simulink model "DTU_Topology_Rural"  (R2023b)
settings: Solver=ode4  StartTime=0.0  StopTime=stoptime  FixedStep=Ts  RelTol=1e-3
PreLoadFcn:
  | Ts=1e-4;load('RuralCase_11052022_12052022_Data_with_ParThreads_Final.mat');run('line_parameters.m');run('Grid_Parameters_3ph.m');
PostLoadFcn:
  | Ts=1e-4;load('RuralCase_11052022_12052022_Data_with_ParThreads_Final.mat');run('line_parameters.m');run('Grid_Parameters_3ph.m');
InitFcn:
  | Ts=1e-4;load('RuralCase_11052022_12052022_Data_with_ParThreads_Final.mat');run('line_parameters.m');run('Grid_Parameters_3ph.m');
StartFcn:
  | Ts=1e-4;load('RuralCase_11052022_12052022_Data_with_ParThreads_Final.mat');run('line_parameters.m');run('Grid_Parameters_3ph.m');
values from neighbouring files (symbols this model uses):
  datastart = 1    [Grid_Parameters_3ph.m]
  datastop = 21556    [Grid_Parameters_3ph.m]
  DTUsignconv = -1000    [Grid_Parameters_3ph.m]
  fnom = 50    [Grid_Parameters_3ph.m]    (also in line_parameters.m)
  line_param = struct()    [line_parameters.m]
  Time = cumsum([0;ones(stoptime,1)])    [Grid_Parameters_3ph.m]
  timestep_meas_data = 1    [Grid_Parameters_3ph.m]
  Vnom = 400    [Grid_Parameters_3ph.m]
undefined symbols (not defined in the file or in its folder): another_event_name, data, j, my_event_name, Newton, Raphson, t_factor
libraries: spsSeriesRLCBranchLib x126, spsGroundLib x71, spsThreePhaseSineGeneratorLib x42, spsControlledCurrentSourceLib x39, spsThreePhaseVIMeasurementLib x26, spsMeanLib x24, spsPowerLib x14, spsMutualInductanceLib x7, rtlab x3, powerlib_meascontrol x3, spsControlledVoltageSourceLib x3, spsThreePhaseSourceLib x1
(part 2 of 5)

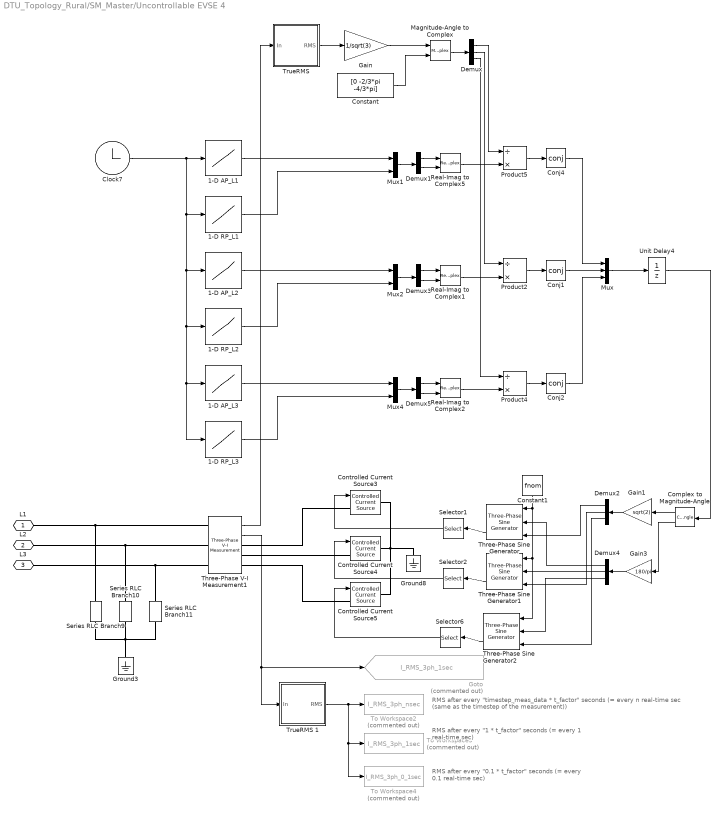
== system DTU_Topology_Rural/SM_Master/Uncontrollable EVSE 4 ==
  note: RMS after every "1 * t_factor" seconds
      | (= every 1 real-time sec)
  note: RMS after every "0.1 * t_factor" seconds
      | (= every 0.1 real-time sec)
  note: RMS after every "timestep_meas_data * t_factor" seconds
      | (= every n real-time sec (same as the timestep of the measurement))
  1-D AP_L1 : Lookup_n-D  NumberOfTableDimensions=1  BreakpointsForDimension1=Time  Table="data.(\"117-6_NEVIC4_phaseA_ActivePower\")(datastart:datastop) * DTUsignconv"  InterpMethod=Flat  InternalRulePriority=Speed  RndMeth=Simplest
  1-D AP_L2 : Lookup_n-D  NumberOfTableDimensions=1  BreakpointsForDimension1=Time  Table="data.(\"117-6_NEVIC4_phaseB_ActivePower\")(datastart:datastop) * DTUsignconv"  InterpMethod=Flat  InternalRulePriority=Speed  RndMeth=Simplest
  1-D AP_L3 : Lookup_n-D  NumberOfTableDimensions=1  BreakpointsForDimension1=Time  Table="data.(\"117-6_NEVIC4_phaseC_ActivePower\")(datastart:datastop) * DTUsignconv"  InterpMethod=Flat  InternalRulePriority=Speed  RndMeth=Simplest
  1-D RP_L1 : Lookup_n-D  NumberOfTableDimensions=1  BreakpointsForDimension1=Time  Table="data.(\"117-6_NEVIC4_phaseA_ReactivePower\")(datastart:datastop) * DTUsignconv"  InterpMethod=Flat  InternalRulePriority=Speed  RndMeth=Simplest
  1-D RP_L2 : Lookup_n-D  NumberOfTableDimensions=1  BreakpointsForDimension1=Time  Table="data.(\"117-6_NEVIC4_phaseB_ReactivePower\")(datastart:datastop) * DTUsignconv"  InterpMethod=Flat  InternalRulePriority=Speed  RndMeth=Simplest
  1-D RP_L3 : Lookup_n-D  NumberOfTableDimensions=1  BreakpointsForDimension1=Time  Table="data.(\"117-6_NEVIC4_phaseC_ReactivePower\")(datastart:datastop) * DTUsignconv"  InterpMethod=Flat  InternalRulePriority=Speed  RndMeth=Simplest
  Clock7 : Clock
  Complex to Magnitude-Angle : ComplexToMagnitudeAngle
  Conj1 : Math  Operator=conj  SignedPower=on
  Conj2 : Math  Operator=conj  SignedPower=on
  Conj4 : Math  Operator=conj  SignedPower=on
  Constant : Constant  Value=[0 -2/3*pi -4/3*pi]
  Constant1 : Constant  Value=fnom
  Controlled Current Source3 : spsControlledCurrentSourceLib/Controlled Current Source  Initialize=on  Source_Type=AC  Amplitude=0  Phase=0  Frequency=50  Measurements=Current
  Controlled Current Source4 : spsControlledCurrentSourceLib/Controlled Current Source  Initialize=on  Source_Type=AC  Amplitude=0  Phase=0  Frequency=50  Measurements=Current
  Controlled Current Source5 : spsControlledCurrentSourceLib/Controlled Current Source  Initialize=on  Source_Type=AC  Amplitude=0  Phase=0  Frequency=50  Measurements=Current
  Demux : Demux  Outputs=3
  Demux1 : Demux  Outputs=2
      settings: DisplayOption=none
  Demux2 : Demux  Outputs=3
  Demux3 : Demux  Outputs=2
      settings: DisplayOption=none
  Demux4 : Demux  Outputs=3
  Demux5 : Demux  Outputs=2
      settings: DisplayOption=none
  Gain : Gain  Gain=1/sqrt(3)
  Gain1 : Gain  Gain=sqrt(2)
  Gain3 : Gain  Gain=180/pi
  Goto : Goto  Commented=on  GotoTag=I_RMS_3ph_1sec  TagVisibility=global
  Ground3 : spsGroundLib/Ground  LConnTagsString=a
  Ground8 : spsGroundLib/Ground  LConnTagsString=a
  Magnitude-Angle to Complex : MagnitudeAngleToComplex
  Mux : Mux  Inputs=3
  Mux1 : Mux  Inputs=2
  Mux2 : Mux  Inputs=2
  Mux4 : Mux  Inputs=2
  Product2 : Product  Inputs=/*  InputSameDT=on  SaturateOnIntegerOverflow=on  OutDataTypeStr=Inherit: Same as first input
  Product4 : Product  Inputs=/*  InputSameDT=on  SaturateOnIntegerOverflow=on  OutDataTypeStr=Inherit: Same as first input
  Product5 : Product  Inputs=/*  InputSameDT=on  SaturateOnIntegerOverflow=on  OutDataTypeStr=Inherit: Same as first input
  Real-Imag to Complex1 : RealImagToComplex
  Real-Imag to Complex2 : RealImagToComplex
  Real-Imag to Complex5 : RealImagToComplex
  Selector1 : Selector  InputPortWidth=3  IndexOptions=Index vector (dialog)  Indices=1  OutputSizes=1
  Selector2 : Selector  InputPortWidth=3  IndexOptions=Index vector (dialog)  Indices=1  OutputSizes=1
  Selector6 : Selector  InputPortWidth=3  IndexOptions=Index vector (dialog)  Indices=1  OutputSizes=1
  Series RLC Branch10 : spsSeriesRLCBranchLib/Series RLC Branch  LConnTagsString=__new0  RConnTagsString=__new0  BranchType=R  Resistance=1e12  Inductance=1e-3  SetiL0=off  InitialCurrent=0  Capacitance=1e-6  Setx0=off  InitialVoltage=0  Measurements=None
  Series RLC Branch11 : spsSeriesRLCBranchLib/Series RLC Branch  LConnTagsString=__new0  RConnTagsString=__new0  BranchType=R  Resistance=1e12  Inductance=1e-3  SetiL0=off  InitialCurrent=0  Capacitance=1e-6  Setx0=off  InitialVoltage=0  Measurements=None
  Series RLC Branch9 : spsSeriesRLCBranchLib/Series RLC Branch  LConnTagsString=__new0  RConnTagsString=__new0  BranchType=R  Resistance=1e12  Inductance=1e-3  SetiL0=off  InitialCurrent=0  Capacitance=1e-6  Setx0=off  InitialVoltage=0  Measurements=None
  Three-Phase Sine Generator : spsThreePhaseSineGeneratorLib/Three-Phase Sine Generator  Ts=0
      settings: LibrarySourceBlock=|
      | sps_lib/Sources/Signal Generator Sources/Three-Phase
      | Sine Generator
  Three-Phase Sine Generator1 : spsThreePhaseSineGeneratorLib/Three-Phase Sine Generator  Ts=0
      settings: LibrarySourceBlock=|
      | sps_lib/Sources/Signal Generator Sources/Three-Phase
      | Sine Generator
  Three-Phase Sine Generator2 : spsThreePhaseSineGeneratorLib/Three-Phase Sine Generator  Ts=0
      settings: LibrarySourceBlock=|
      | sps_lib/Sources/Signal Generator Sources/Three-Phase
      | Sine Generator
  Three-Phase V-I Measurement1 : spsThreePhaseVIMeasurementLib/Three-Phase V-I Measurement  VoltageMeasurement=phase-to-phase  SetLabelV=off  LabelV=Vabc  Vpu=off  VpuLL=off  CurrentMeasurement=yes  SetLabelI=off  LabelI=Iabc  Ipu=off  Pbase=100e6  Vbase=Vnom*sqrt(3)  OutputType=Complex  PhasorSimulation=off  PSBequivalent=0
  To Workspace2 : ToWorkspace  Commented=on  VariableName=I_RMS_3ph_nsec  SampleTime=timestep_meas_data * t_factor
  To Workspace4 : ToWorkspace  Commented=on  VariableName=I_RMS_3ph_0_1sec  SampleTime=0.1 * t_factor
  To Workspace5 : ToWorkspace  Commented=on  VariableName=I_RMS_3ph_1sec  SampleTime=1 * t_factor
  "TrueRMS " : Subsystem  AncestorBlock=powerlib_meascontrol/Measurements/RMS/TrueRMS
  TrueRMS 1 : Subsystem  AncestorBlock=powerlib_meascontrol/Measurements/RMS/TrueRMS
  Unit Delay4 : UnitDelay  InitialCondition=0*exp(-j*0*pi/180)  SampleTime=Ts  HasFrameUpgradeWarning=on
  L1 : PMIOPort  Side=Right
  L2 : PMIOPort  Port=2  Side=Right
  L3 : PMIOPort  Port=3  Side=Right
  wires:
  1-D AP_L1/1 -> Mux1/1
  Product5/1 -> Conj4/1
  Three-Phase V-I Measurement1/2 -> Goto/1, TrueRMS 1/1(In)
  Mux1/1 -> Demux1/1
  Real-Imag to Complex5/1 -> Product5/2
  Clock7/1 -> 1-D RP_L1/1, 1-D RP_L2/1, 1-D AP_L3/1, 1-D RP_L3/1, 1-D AP_L2/1, 1-D AP_L1/1
  TrueRMS 1/1(RMS) -> To Workspace2/1, To Workspace5/1, To Workspace4/1
  Constant/1 -> Magnitude-Angle to Complex/2
  Demux/1 -> Product5/1
  Demux/2 -> Product2/1
  Demux/3 -> Product4/1
  Magnitude-Angle to Complex/1 -> Demux/1
  Gain/1 -> Magnitude-Angle to Complex/1
  Mux/1 -> Unit Delay4/1
  Complex to Magnitude-Angle/1 -> Gain1/1
  Three-Phase Sine Generator/1 -> Selector1/1
  Three-Phase Sine Generator1/1 -> Selector2/1
  Three-Phase Sine Generator2/1 -> Selector6/1
  Selector2/1 -> Controlled Current Source4/1
  Selector6/1 -> Controlled Current Source5/1
  Demux2/1 -> Three-Phase Sine Generator/1
  Demux2/2 -> Three-Phase Sine Generator1/1
  Demux2/3 -> Three-Phase Sine Generator2/1
  Conj4/1 -> Mux/1
  Conj1/1 -> Mux/2
  Conj2/1 -> Mux/3
  Constant1/1 -> Three-Phase Sine Generator/3, Three-Phase Sine Generator2/3, Three-Phase Sine Generator1/3
  Complex to Magnitude-Angle/2 -> Gain3/1
  Gain3/1 -> Demux4/1
  Selector1/1 -> Controlled Current Source3/1
  Demux4/1 -> Three-Phase Sine Generator/2
  Demux4/2 -> Three-Phase Sine Generator1/2
  Demux4/3 -> Three-Phase Sine Generator2/2
  Gain1/1 -> Demux2/1
  Demux1/1 -> Real-Imag to Complex5/1
  Demux1/2 -> Real-Imag to Complex5/2
  "TrueRMS "/1(RMS) -> Gain/1
  Three-Phase V-I Measurement1/1 -> "TrueRMS "/1(In)
  Unit Delay4/1 -> Complex to Magnitude-Angle/1
  Mux2/1 -> Demux3/1
  Demux3/2 -> Real-Imag to Complex1/2
  Real-Imag to Complex1/1 -> Product2/2
  Demux3/1 -> Real-Imag to Complex1/1
  1-D AP_L2/1 -> Mux2/1
  Product2/1 -> Conj1/1
  Mux4/1 -> Demux5/1
  Demux5/2 -> Real-Imag to Complex2/2
  Real-Imag to Complex2/1 -> Product4/2
  Demux5/1 -> Real-Imag to Complex2/1
  1-D AP_L3/1 -> Mux4/1
  Product4/1 -> Conj2/1
  1-D RP_L1/1 -> Mux1/2
  1-D RP_L2/1 -> Mux2/2
  1-D RP_L3/1 -> Mux4/2
  connections:
  Three-Phase V-I Measurement1/RConn2 -- Controlled Current Source4/LConn1
  Three-Phase V-I Measurement1/RConn1 -- Controlled Current Source3/LConn1
  Three-Phase V-I Measurement1/RConn3 -- Controlled Current Source5/LConn1
  Controlled Current Source3/RConn1 -- Controlled Current Source4/RConn1 -- Ground8/LConn1 -- Controlled Current Source5/RConn1
  L1/RConn1 -- Three-Phase V-I Measurement1/LConn1 -- Series RLC Branch9/LConn1
  Series RLC Branch10/LConn1 -- Three-Phase V-I Measurement1/LConn2 -- L2/RConn1
  Series RLC Branch11/LConn1 -- Three-Phase V-I Measurement1/LConn3 -- L3/RConn1
  Series RLC Branch9/RConn1 -- Series RLC Branch10/RConn1 -- Ground3/LConn1 -- Series RLC Branch11/RConn1

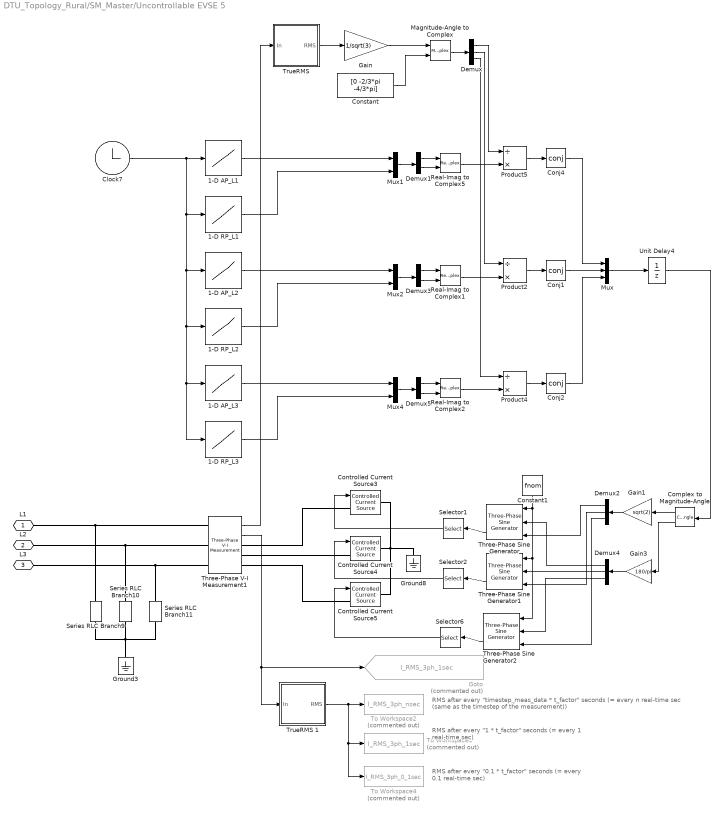
== system DTU_Topology_Rural/SM_Master/Uncontrollable EVSE 5 ==
  note: RMS after every "1 * t_factor" seconds
      | (= every 1 real-time sec)
  note: RMS after every "0.1 * t_factor" seconds
      | (= every 0.1 real-time sec)
  note: RMS after every "timestep_meas_data * t_factor" seconds
      | (= every n real-time sec (same as the timestep of the measurement))
  1-D AP_L1 : Lookup_n-D  NumberOfTableDimensions=1  BreakpointsForDimension1=Time  Table="data.(\"117-6_NEVIC5_phaseA_ActivePower\")(datastart:datastop) * DTUsignconv"  InterpMethod=Flat  InternalRulePriority=Speed  RndMeth=Simplest
  1-D AP_L2 : Lookup_n-D  NumberOfTableDimensions=1  BreakpointsForDimension1=Time  Table="data.(\"117-6_NEVIC5_phaseB_ActivePower\")(datastart:datastop) * DTUsignconv"  InterpMethod=Flat  InternalRulePriority=Speed  RndMeth=Simplest
  1-D AP_L3 : Lookup_n-D  NumberOfTableDimensions=1  BreakpointsForDimension1=Time  Table="data.(\"117-6_NEVIC5_phaseC_ActivePower\")(datastart:datastop) * DTUsignconv"  InterpMethod=Flat  InternalRulePriority=Speed  RndMeth=Simplest
  1-D RP_L1 : Lookup_n-D  NumberOfTableDimensions=1  BreakpointsForDimension1=Time  Table="data.(\"117-6_NEVIC5_phaseA_ReactivePower\")(datastart:datastop) * DTUsignconv"  InterpMethod=Flat  InternalRulePriority=Speed  RndMeth=Simplest
  1-D RP_L2 : Lookup_n-D  NumberOfTableDimensions=1  BreakpointsForDimension1=Time  Table="data.(\"117-6_NEVIC5_phaseB_ReactivePower\")(datastart:datastop) * DTUsignconv"  InterpMethod=Flat  InternalRulePriority=Speed  RndMeth=Simplest
  1-D RP_L3 : Lookup_n-D  NumberOfTableDimensions=1  BreakpointsForDimension1=Time  Table="data.(\"117-6_NEVIC5_phaseC_ReactivePower\")(datastart:datastop) * DTUsignconv"  InterpMethod=Flat  InternalRulePriority=Speed  RndMeth=Simplest
  Clock7 : Clock
  Complex to Magnitude-Angle : ComplexToMagnitudeAngle
  Conj1 : Math  Operator=conj  SignedPower=on
  Conj2 : Math  Operator=conj  SignedPower=on
  Conj4 : Math  Operator=conj  SignedPower=on
  Constant : Constant  Value=[0 -2/3*pi -4/3*pi]
  Constant1 : Constant  Value=fnom
  Controlled Current Source3 : spsControlledCurrentSourceLib/Controlled Current Source  Initialize=on  Source_Type=AC  Amplitude=0  Phase=0  Frequency=50  Measurements=Current
  Controlled Current Source4 : spsControlledCurrentSourceLib/Controlled Current Source  Initialize=on  Source_Type=AC  Amplitude=0  Phase=0  Frequency=50  Measurements=Current
  Controlled Current Source5 : spsControlledCurrentSourceLib/Controlled Current Source  Initialize=on  Source_Type=AC  Amplitude=0  Phase=0  Frequency=50  Measurements=Current
  Demux : Demux  Outputs=3
  Demux1 : Demux  Outputs=2
      settings: DisplayOption=none
  Demux2 : Demux  Outputs=3
  Demux3 : Demux  Outputs=2
      settings: DisplayOption=none
  Demux4 : Demux  Outputs=3
  Demux5 : Demux  Outputs=2
      settings: DisplayOption=none
  Gain : Gain  Gain=1/sqrt(3)
  Gain1 : Gain  Gain=sqrt(2)
  Gain3 : Gain  Gain=180/pi
  Goto : Goto  Commented=on  GotoTag=I_RMS_3ph_1sec  TagVisibility=global
  Ground3 : spsGroundLib/Ground  LConnTagsString=a
  Ground8 : spsGroundLib/Ground  LConnTagsString=a
  Magnitude-Angle to Complex : MagnitudeAngleToComplex
  Mux : Mux  Inputs=3
  Mux1 : Mux  Inputs=2
  Mux2 : Mux  Inputs=2
  Mux4 : Mux  Inputs=2
  Product2 : Product  Inputs=/*  InputSameDT=on  SaturateOnIntegerOverflow=on  OutDataTypeStr=Inherit: Same as first input
  Product4 : Product  Inputs=/*  InputSameDT=on  SaturateOnIntegerOverflow=on  OutDataTypeStr=Inherit: Same as first input
  Product5 : Product  Inputs=/*  InputSameDT=on  SaturateOnIntegerOverflow=on  OutDataTypeStr=Inherit: Same as first input
  Real-Imag to Complex1 : RealImagToComplex
  Real-Imag to Complex2 : RealImagToComplex
  Real-Imag to Complex5 : RealImagToComplex
  Selector1 : Selector  InputPortWidth=3  IndexOptions=Index vector (dialog)  Indices=1  OutputSizes=1
  Selector2 : Selector  InputPortWidth=3  IndexOptions=Index vector (dialog)  Indices=1  OutputSizes=1
  Selector6 : Selector  InputPortWidth=3  IndexOptions=Index vector (dialog)  Indices=1  OutputSizes=1
  Series RLC Branch10 : spsSeriesRLCBranchLib/Series RLC Branch  LConnTagsString=__new0  RConnTagsString=__new0  BranchType=R  Resistance=1e12  Inductance=1e-3  SetiL0=off  InitialCurrent=0  Capacitance=1e-6  Setx0=off  InitialVoltage=0  Measurements=None
  Series RLC Branch11 : spsSeriesRLCBranchLib/Series RLC Branch  LConnTagsString=__new0  RConnTagsString=__new0  BranchType=R  Resistance=1e12  Inductance=1e-3  SetiL0=off  InitialCurrent=0  Capacitance=1e-6  Setx0=off  InitialVoltage=0  Measurements=None
  Series RLC Branch9 : spsSeriesRLCBranchLib/Series RLC Branch  LConnTagsString=__new0  RConnTagsString=__new0  BranchType=R  Resistance=1e12  Inductance=1e-3  SetiL0=off  InitialCurrent=0  Capacitance=1e-6  Setx0=off  InitialVoltage=0  Measurements=None
  Three-Phase Sine Generator : spsThreePhaseSineGeneratorLib/Three-Phase Sine Generator  Ts=0
      settings: LibrarySourceBlock=|
      | sps_lib/Sources/Signal Generator Sources/Three-Phase
      | Sine Generator
  Three-Phase Sine Generator1 : spsThreePhaseSineGeneratorLib/Three-Phase Sine Generator  Ts=0
      settings: LibrarySourceBlock=|
      | sps_lib/Sources/Signal Generator Sources/Three-Phase
      | Sine Generator
  Three-Phase Sine Generator2 : spsThreePhaseSineGeneratorLib/Three-Phase Sine Generator  Ts=0
      settings: LibrarySourceBlock=|
      | sps_lib/Sources/Signal Generator Sources/Three-Phase
      | Sine Generator
  Three-Phase V-I Measurement1 : spsThreePhaseVIMeasurementLib/Three-Phase V-I Measurement  VoltageMeasurement=phase-to-phase  SetLabelV=off  LabelV=Vabc  Vpu=off  VpuLL=off  CurrentMeasurement=yes  SetLabelI=off  LabelI=Iabc  Ipu=off  Pbase=100e6  Vbase=Vnom*sqrt(3)  OutputType=Complex  PhasorSimulation=off  PSBequivalent=0
  To Workspace2 : ToWorkspace  Commented=on  VariableName=I_RMS_3ph_nsec  SampleTime=timestep_meas_data * t_factor
  To Workspace4 : ToWorkspace  Commented=on  VariableName=I_RMS_3ph_0_1sec  SampleTime=0.1 * t_factor
  To Workspace5 : ToWorkspace  Commented=on  VariableName=I_RMS_3ph_1sec  SampleTime=1 * t_factor
  "TrueRMS " : Subsystem  AncestorBlock=powerlib_meascontrol/Measurements/RMS/TrueRMS
  TrueRMS 1 : Subsystem  AncestorBlock=powerlib_meascontrol/Measurements/RMS/TrueRMS
  Unit Delay4 : UnitDelay  InitialCondition=0*exp(-j*0*pi/180)  SampleTime=Ts  HasFrameUpgradeWarning=on
  L1 : PMIOPort  Side=Right
  L2 : PMIOPort  Port=2  Side=Right
  L3 : PMIOPort  Port=3  Side=Right
  wires:
  1-D AP_L1/1 -> Mux1/1
  Product5/1 -> Conj4/1
  Three-Phase V-I Measurement1/2 -> Goto/1, TrueRMS 1/1(In)
  Mux1/1 -> Demux1/1
  Real-Imag to Complex5/1 -> Product5/2
  Clock7/1 -> 1-D RP_L1/1, 1-D RP_L2/1, 1-D AP_L3/1, 1-D RP_L3/1, 1-D AP_L2/1, 1-D AP_L1/1
  TrueRMS 1/1(RMS) -> To Workspace2/1, To Workspace5/1, To Workspace4/1
  Constant/1 -> Magnitude-Angle to Complex/2
  Demux/1 -> Product5/1
  Demux/2 -> Product2/1
  Demux/3 -> Product4/1
  Magnitude-Angle to Complex/1 -> Demux/1
  Gain/1 -> Magnitude-Angle to Complex/1
  Mux/1 -> Unit Delay4/1
  Complex to Magnitude-Angle/1 -> Gain1/1
  Three-Phase Sine Generator/1 -> Selector1/1
  Three-Phase Sine Generator1/1 -> Selector2/1
  Three-Phase Sine Generator2/1 -> Selector6/1
  Selector2/1 -> Controlled Current Source4/1
  Selector6/1 -> Controlled Current Source5/1
  Demux2/1 -> Three-Phase Sine Generator/1
  Demux2/2 -> Three-Phase Sine Generator1/1
  Demux2/3 -> Three-Phase Sine Generator2/1
  Conj4/1 -> Mux/1
  Conj1/1 -> Mux/2
  Conj2/1 -> Mux/3
  Constant1/1 -> Three-Phase Sine Generator/3, Three-Phase Sine Generator2/3, Three-Phase Sine Generator1/3
  Complex to Magnitude-Angle/2 -> Gain3/1
  Gain3/1 -> Demux4/1
  Selector1/1 -> Controlled Current Source3/1
  Demux4/1 -> Three-Phase Sine Generator/2
  Demux4/2 -> Three-Phase Sine Generator1/2
  Demux4/3 -> Three-Phase Sine Generator2/2
  Gain1/1 -> Demux2/1
  Demux1/1 -> Real-Imag to Complex5/1
  Demux1/2 -> Real-Imag to Complex5/2
  "TrueRMS "/1(RMS) -> Gain/1
  Three-Phase V-I Measurement1/1 -> "TrueRMS "/1(In)
  Unit Delay4/1 -> Complex to Magnitude-Angle/1
  Mux2/1 -> Demux3/1
  Demux3/2 -> Real-Imag to Complex1/2
  Real-Imag to Complex1/1 -> Product2/2
  Demux3/1 -> Real-Imag to Complex1/1
  1-D AP_L2/1 -> Mux2/1
  Product2/1 -> Conj1/1
  Mux4/1 -> Demux5/1
  Demux5/2 -> Real-Imag to Complex2/2
  Real-Imag to Complex2/1 -> Product4/2
  Demux5/1 -> Real-Imag to Complex2/1
  1-D AP_L3/1 -> Mux4/1
  Product4/1 -> Conj2/1
  1-D RP_L1/1 -> Mux1/2
  1-D RP_L2/1 -> Mux2/2
  1-D RP_L3/1 -> Mux4/2
  connections:
  Three-Phase V-I Measurement1/RConn2 -- Controlled Current Source4/LConn1
  Three-Phase V-I Measurement1/RConn1 -- Controlled Current Source3/LConn1
  Three-Phase V-I Measurement1/RConn3 -- Controlled Current Source5/LConn1
  Controlled Current Source3/RConn1 -- Controlled Current Source4/RConn1 -- Ground8/LConn1 -- Controlled Current Source5/RConn1
  L1/RConn1 -- Three-Phase V-I Measurement1/LConn1 -- Series RLC Branch9/LConn1
  Series RLC Branch10/LConn1 -- Three-Phase V-I Measurement1/LConn2 -- L2/RConn1
  Series RLC Branch11/LConn1 -- Three-Phase V-I Measurement1/LConn3 -- L3/RConn1
  Series RLC Branch9/RConn1 -- Series RLC Branch10/RConn1 -- Ground3/LConn1 -- Series RLC Branch11/RConn1

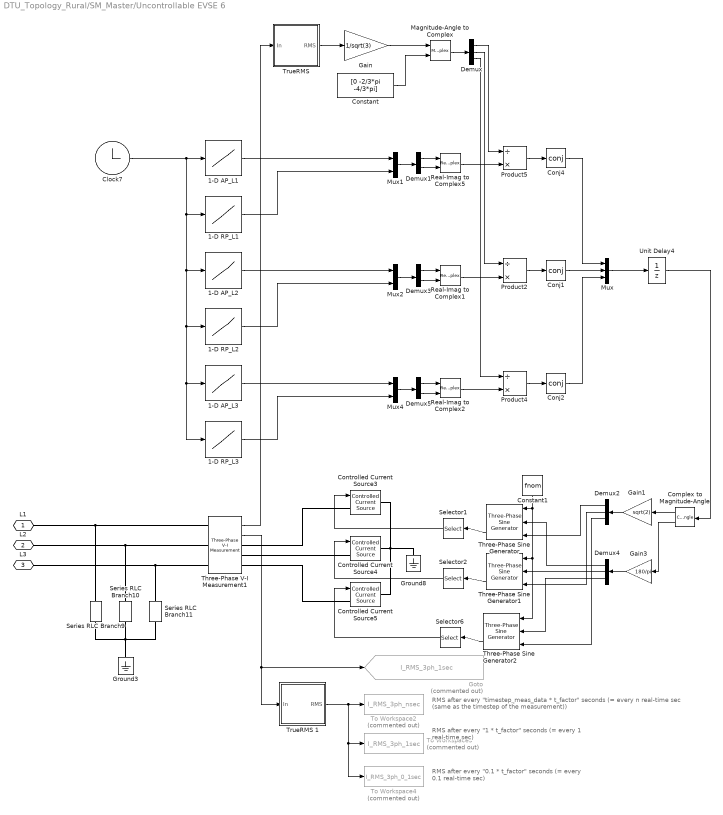
== system DTU_Topology_Rural/SM_Master/Uncontrollable EVSE 6 ==
  note: RMS after every "1 * t_factor" seconds
      | (= every 1 real-time sec)
  note: RMS after every "0.1 * t_factor" seconds
      | (= every 0.1 real-time sec)
  note: RMS after every "timestep_meas_data * t_factor" seconds
      | (= every n real-time sec (same as the timestep of the measurement))
  1-D AP_L1 : Lookup_n-D  NumberOfTableDimensions=1  BreakpointsForDimension1=Time  Table="data.(\"117-6_NEVIC6_phaseA_ActivePower\")(datastart:datastop) * DTUsignconv"  InterpMethod=Flat  InternalRulePriority=Speed  RndMeth=Simplest
  1-D AP_L2 : Lookup_n-D  NumberOfTableDimensions=1  BreakpointsForDimension1=Time  Table="data.(\"117-6_NEVIC6_phaseB_ActivePower\")(datastart:datastop) * DTUsignconv"  InterpMethod=Flat  InternalRulePriority=Speed  RndMeth=Simplest
  1-D AP_L3 : Lookup_n-D  NumberOfTableDimensions=1  BreakpointsForDimension1=Time  Table="data.(\"117-6_NEVIC6_phaseC_ActivePower\")(datastart:datastop) * DTUsignconv"  InterpMethod=Flat  InternalRulePriority=Speed  RndMeth=Simplest
  1-D RP_L1 : Lookup_n-D  NumberOfTableDimensions=1  BreakpointsForDimension1=Time  Table="data.(\"117-6_NEVIC6_phaseA_ReactivePower\")(datastart:datastop) * DTUsignconv"  InterpMethod=Flat  InternalRulePriority=Speed  RndMeth=Simplest
  1-D RP_L2 : Lookup_n-D  NumberOfTableDimensions=1  BreakpointsForDimension1=Time  Table="data.(\"117-6_NEVIC6_phaseB_ReactivePower\")(datastart:datastop) * DTUsignconv"  InterpMethod=Flat  InternalRulePriority=Speed  RndMeth=Simplest
  1-D RP_L3 : Lookup_n-D  NumberOfTableDimensions=1  BreakpointsForDimension1=Time  Table="data.(\"117-6_NEVIC6_phaseC_ReactivePower\")(datastart:datastop) * DTUsignconv"  InterpMethod=Flat  InternalRulePriority=Speed  RndMeth=Simplest
  Clock7 : Clock
  Complex to Magnitude-Angle : ComplexToMagnitudeAngle
  Conj1 : Math  Operator=conj  SignedPower=on
  Conj2 : Math  Operator=conj  SignedPower=on
  Conj4 : Math  Operator=conj  SignedPower=on
  Constant : Constant  Value=[0 -2/3*pi -4/3*pi]
  Constant1 : Constant  Value=fnom
  Controlled Current Source3 : spsControlledCurrentSourceLib/Controlled Current Source  Initialize=on  Source_Type=AC  Amplitude=0  Phase=0  Frequency=50  Measurements=Current
  Controlled Current Source4 : spsControlledCurrentSourceLib/Controlled Current Source  Initialize=on  Source_Type=AC  Amplitude=0  Phase=0  Frequency=50  Measurements=Current
  Controlled Current Source5 : spsControlledCurrentSourceLib/Controlled Current Source  Initialize=on  Source_Type=AC  Amplitude=0  Phase=0  Frequency=50  Measurements=Current
  Demux : Demux  Outputs=3
  Demux1 : Demux  Outputs=2
      settings: DisplayOption=none
  Demux2 : Demux  Outputs=3
  Demux3 : Demux  Outputs=2
      settings: DisplayOption=none
  Demux4 : Demux  Outputs=3
  Demux5 : Demux  Outputs=2
      settings: DisplayOption=none
  Gain : Gain  Gain=1/sqrt(3)
  Gain1 : Gain  Gain=sqrt(2)
  Gain3 : Gain  Gain=180/pi
  Goto : Goto  Commented=on  GotoTag=I_RMS_3ph_1sec  TagVisibility=global
  Ground3 : spsGroundLib/Ground  LConnTagsString=a
  Ground8 : spsGroundLib/Ground  LConnTagsString=a
  Magnitude-Angle to Complex : MagnitudeAngleToComplex
  Mux : Mux  Inputs=3
  Mux1 : Mux  Inputs=2
  Mux2 : Mux  Inputs=2
  Mux4 : Mux  Inputs=2
  Product2 : Product  Inputs=/*  InputSameDT=on  SaturateOnIntegerOverflow=on  OutDataTypeStr=Inherit: Same as first input
  Product4 : Product  Inputs=/*  InputSameDT=on  SaturateOnIntegerOverflow=on  OutDataTypeStr=Inherit: Same as first input
  Product5 : Product  Inputs=/*  InputSameDT=on  SaturateOnIntegerOverflow=on  OutDataTypeStr=Inherit: Same as first input
  Real-Imag to Complex1 : RealImagToComplex
  Real-Imag to Complex2 : RealImagToComplex
  Real-Imag to Complex5 : RealImagToComplex
  Selector1 : Selector  InputPortWidth=3  IndexOptions=Index vector (dialog)  Indices=1  OutputSizes=1
  Selector2 : Selector  InputPortWidth=3  IndexOptions=Index vector (dialog)  Indices=1  OutputSizes=1
  Selector6 : Selector  InputPortWidth=3  IndexOptions=Index vector (dialog)  Indices=1  OutputSizes=1
  Series RLC Branch10 : spsSeriesRLCBranchLib/Series RLC Branch  LConnTagsString=__new0  RConnTagsString=__new0  BranchType=R  Resistance=1e12  Inductance=1e-3  SetiL0=off  InitialCurrent=0  Capacitance=1e-6  Setx0=off  InitialVoltage=0  Measurements=None
  Series RLC Branch11 : spsSeriesRLCBranchLib/Series RLC Branch  LConnTagsString=__new0  RConnTagsString=__new0  BranchType=R  Resistance=1e12  Inductance=1e-3  SetiL0=off  InitialCurrent=0  Capacitance=1e-6  Setx0=off  InitialVoltage=0  Measurements=None
  Series RLC Branch9 : spsSeriesRLCBranchLib/Series RLC Branch  LConnTagsString=__new0  RConnTagsString=__new0  BranchType=R  Resistance=1e12  Inductance=1e-3  SetiL0=off  InitialCurrent=0  Capacitance=1e-6  Setx0=off  InitialVoltage=0  Measurements=None
  Three-Phase Sine Generator : spsThreePhaseSineGeneratorLib/Three-Phase Sine Generator  Ts=0
      settings: LibrarySourceBlock=|
      | sps_lib/Sources/Signal Generator Sources/Three-Phase
      | Sine Generator
  Three-Phase Sine Generator1 : spsThreePhaseSineGeneratorLib/Three-Phase Sine Generator  Ts=0
      settings: LibrarySourceBlock=|
      | sps_lib/Sources/Signal Generator Sources/Three-Phase
      | Sine Generator
  Three-Phase Sine Generator2 : spsThreePhaseSineGeneratorLib/Three-Phase Sine Generator  Ts=0
      settings: LibrarySourceBlock=|
      | sps_lib/Sources/Signal Generator Sources/Three-Phase
      | Sine Generator
  Three-Phase V-I Measurement1 : spsThreePhaseVIMeasurementLib/Three-Phase V-I Measurement  VoltageMeasurement=phase-to-phase  SetLabelV=off  LabelV=Vabc  Vpu=off  VpuLL=off  CurrentMeasurement=yes  SetLabelI=off  LabelI=Iabc  Ipu=off  Pbase=100e6  Vbase=Vnom*sqrt(3)  OutputType=Complex  PhasorSimulation=off  PSBequivalent=0
  To Workspace2 : ToWorkspace  Commented=on  VariableName=I_RMS_3ph_nsec  SampleTime=timestep_meas_data * t_factor
  To Workspace4 : ToWorkspace  Commented=on  VariableName=I_RMS_3ph_0_1sec  SampleTime=0.1 * t_factor
  To Workspace5 : ToWorkspace  Commented=on  VariableName=I_RMS_3ph_1sec  SampleTime=1 * t_factor
  "TrueRMS " : Subsystem  AncestorBlock=powerlib_meascontrol/Measurements/RMS/TrueRMS
  TrueRMS 1 : Subsystem  AncestorBlock=powerlib_meascontrol/Measurements/RMS/TrueRMS
  Unit Delay4 : UnitDelay  InitialCondition=0*exp(-j*0*pi/180)  SampleTime=Ts  HasFrameUpgradeWarning=on
  L1 : PMIOPort  Side=Right
  L2 : PMIOPort  Port=2  Side=Right
  L3 : PMIOPort  Port=3  Side=Right
  wires:
  1-D AP_L1/1 -> Mux1/1
  Product5/1 -> Conj4/1
  Three-Phase V-I Measurement1/2 -> Goto/1, TrueRMS 1/1(In)
  Mux1/1 -> Demux1/1
  Real-Imag to Complex5/1 -> Product5/2
  Clock7/1 -> 1-D RP_L1/1, 1-D RP_L2/1, 1-D AP_L3/1, 1-D RP_L3/1, 1-D AP_L2/1, 1-D AP_L1/1
  TrueRMS 1/1(RMS) -> To Workspace2/1, To Workspace5/1, To Workspace4/1
  Constant/1 -> Magnitude-Angle to Complex/2
  Demux/1 -> Product5/1
  Demux/2 -> Product2/1
  Demux/3 -> Product4/1
  Magnitude-Angle to Complex/1 -> Demux/1
  Gain/1 -> Magnitude-Angle to Complex/1
  Mux/1 -> Unit Delay4/1
  Complex to Magnitude-Angle/1 -> Gain1/1
  Three-Phase Sine Generator/1 -> Selector1/1
  Three-Phase Sine Generator1/1 -> Selector2/1
  Three-Phase Sine Generator2/1 -> Selector6/1
  Selector2/1 -> Controlled Current Source4/1
  Selector6/1 -> Controlled Current Source5/1
  Demux2/1 -> Three-Phase Sine Generator/1
  Demux2/2 -> Three-Phase Sine Generator1/1
  Demux2/3 -> Three-Phase Sine Generator2/1
  Conj4/1 -> Mux/1
  Conj1/1 -> Mux/2
  Conj2/1 -> Mux/3
  Constant1/1 -> Three-Phase Sine Generator/3, Three-Phase Sine Generator2/3, Three-Phase Sine Generator1/3
  Complex to Magnitude-Angle/2 -> Gain3/1
  Gain3/1 -> Demux4/1
  Selector1/1 -> Controlled Current Source3/1
  Demux4/1 -> Three-Phase Sine Generator/2
  Demux4/2 -> Three-Phase Sine Generator1/2
  Demux4/3 -> Three-Phase Sine Generator2/2
  Gain1/1 -> Demux2/1
  Demux1/1 -> Real-Imag to Complex5/1
  Demux1/2 -> Real-Imag to Complex5/2
  "TrueRMS "/1(RMS) -> Gain/1
  Three-Phase V-I Measurement1/1 -> "TrueRMS "/1(In)
  Unit Delay4/1 -> Complex to Magnitude-Angle/1
  Mux2/1 -> Demux3/1
  Demux3/2 -> Real-Imag to Complex1/2
  Real-Imag to Complex1/1 -> Product2/2
  Demux3/1 -> Real-Imag to Complex1/1
  1-D AP_L2/1 -> Mux2/1
  Product2/1 -> Conj1/1
  Mux4/1 -> Demux5/1
  Demux5/2 -> Real-Imag to Complex2/2
  Real-Imag to Complex2/1 -> Product4/2
  Demux5/1 -> Real-Imag to Complex2/1
  1-D AP_L3/1 -> Mux4/1
  Product4/1 -> Conj2/1
  1-D RP_L1/1 -> Mux1/2
  1-D RP_L2/1 -> Mux2/2
  1-D RP_L3/1 -> Mux4/2
  connections:
  Three-Phase V-I Measurement1/RConn2 -- Controlled Current Source4/LConn1
  Three-Phase V-I Measurement1/RConn1 -- Controlled Current Source3/LConn1
  Three-Phase V-I Measurement1/RConn3 -- Controlled Current Source5/LConn1
  Controlled Current Source3/RConn1 -- Controlled Current Source4/RConn1 -- Ground8/LConn1 -- Controlled Current Source5/RConn1
  L1/RConn1 -- Three-Phase V-I Measurement1/LConn1 -- Series RLC Branch9/LConn1
  Series RLC Branch10/LConn1 -- Three-Phase V-I Measurement1/LConn2 -- L2/RConn1
  Series RLC Branch11/LConn1 -- Three-Phase V-I Measurement1/LConn3 -- L3/RConn1
  Series RLC Branch9/RConn1 -- Series RLC Branch10/RConn1 -- Ground3/LConn1 -- Series RLC Branch11/RConn1

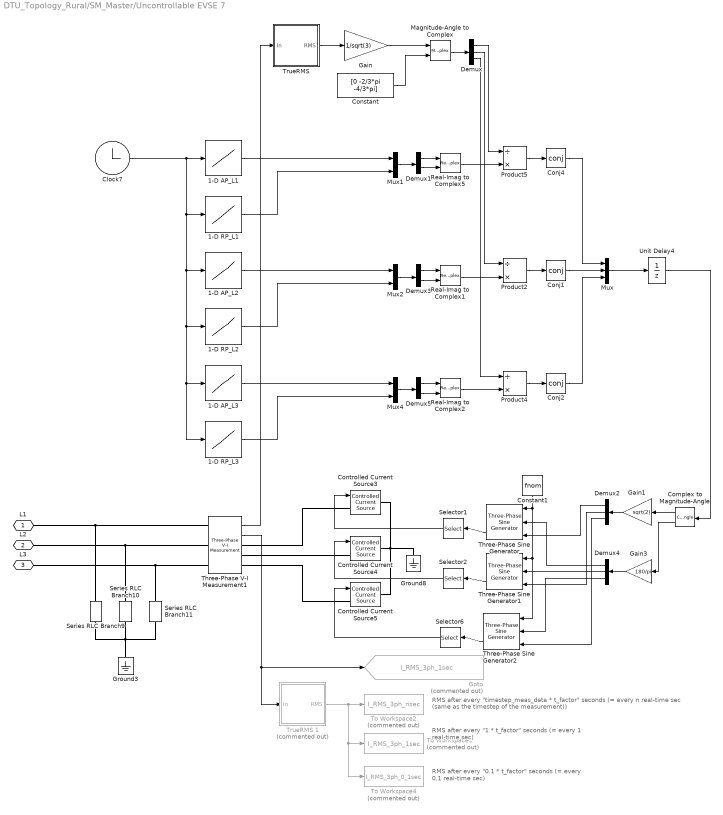
== system DTU_Topology_Rural/SM_Master/Uncontrollable EVSE 7 ==
  note: RMS after every "1 * t_factor" seconds
      | (= every 1 real-time sec)
  note: RMS after every "0.1 * t_factor" seconds
      | (= every 0.1 real-time sec)
  note: RMS after every "timestep_meas_data * t_factor" seconds
      | (= every n real-time sec (same as the timestep of the measurement))
  1-D AP_L1 : Lookup_n-D  NumberOfTableDimensions=1  BreakpointsForDimension1=Time  Table="data.(\"117-6_NEVIC7_phaseA_ActivePower\")(datastart:datastop) * DTUsignconv"  InterpMethod=Flat  InternalRulePriority=Speed  RndMeth=Simplest
  1-D AP_L2 : Lookup_n-D  NumberOfTableDimensions=1  BreakpointsForDimension1=Time  Table="data.(\"117-6_NEVIC7_phaseB_ActivePower\")(datastart:datastop) * DTUsignconv"  InterpMethod=Flat  InternalRulePriority=Speed  RndMeth=Simplest
  1-D AP_L3 : Lookup_n-D  NumberOfTableDimensions=1  BreakpointsForDimension1=Time  Table="data.(\"117-6_NEVIC7_phaseC_ActivePower\")(datastart:datastop) * DTUsignconv"  InterpMethod=Flat  InternalRulePriority=Speed  RndMeth=Simplest
  1-D RP_L1 : Lookup_n-D  NumberOfTableDimensions=1  BreakpointsForDimension1=Time  Table="data.(\"117-6_NEVIC7_phaseA_ReactivePower\")(datastart:datastop) * DTUsignconv"  InterpMethod=Flat  InternalRulePriority=Speed  RndMeth=Simplest
  1-D RP_L2 : Lookup_n-D  NumberOfTableDimensions=1  BreakpointsForDimension1=Time  Table="data.(\"117-6_NEVIC7_phaseB_ReactivePower\")(datastart:datastop) * DTUsignconv"  InterpMethod=Flat  InternalRulePriority=Speed  RndMeth=Simplest
  1-D RP_L3 : Lookup_n-D  NumberOfTableDimensions=1  BreakpointsForDimension1=Time  Table="data.(\"117-6_NEVIC7_phaseC_ReactivePower\")(datastart:datastop) * DTUsignconv"  InterpMethod=Flat  InternalRulePriority=Speed  RndMeth=Simplest
  Clock7 : Clock
  Complex to Magnitude-Angle : ComplexToMagnitudeAngle
  Conj1 : Math  Operator=conj  SignedPower=on
  Conj2 : Math  Operator=conj  SignedPower=on
  Conj4 : Math  Operator=conj  SignedPower=on
  Constant : Constant  Value=[0 -2/3*pi -4/3*pi]
  Constant1 : Constant  Value=fnom
  Controlled Current Source3 : spsControlledCurrentSourceLib/Controlled Current Source  Initialize=on  Source_Type=AC  Amplitude=0  Phase=0  Frequency=50  Measurements=Current
  Controlled Current Source4 : spsControlledCurrentSourceLib/Controlled Current Source  Initialize=on  Source_Type=AC  Amplitude=0  Phase=0  Frequency=50  Measurements=Current
  Controlled Current Source5 : spsControlledCurrentSourceLib/Controlled Current Source  Initialize=on  Source_Type=AC  Amplitude=0  Phase=0  Frequency=50  Measurements=Current
  Demux : Demux  Outputs=3
  Demux1 : Demux  Outputs=2
      settings: DisplayOption=none
  Demux2 : Demux  Outputs=3
  Demux3 : Demux  Outputs=2
      settings: DisplayOption=none
  Demux4 : Demux  Outputs=3
  Demux5 : Demux  Outputs=2
      settings: DisplayOption=none
  Gain : Gain  Gain=1/sqrt(3)
  Gain1 : Gain  Gain=sqrt(2)
  Gain3 : Gain  Gain=180/pi
  Goto : Goto  Commented=on  GotoTag=I_RMS_3ph_1sec  TagVisibility=global
  Ground3 : spsGroundLib/Ground  LConnTagsString=a
  Ground8 : spsGroundLib/Ground  LConnTagsString=a
  Magnitude-Angle to Complex : MagnitudeAngleToComplex
  Mux : Mux  Inputs=3
  Mux1 : Mux  Inputs=2
  Mux2 : Mux  Inputs=2
  Mux4 : Mux  Inputs=2
  Product2 : Product  Inputs=/*  InputSameDT=on  SaturateOnIntegerOverflow=on  OutDataTypeStr=Inherit: Same as first input
  Product4 : Product  Inputs=/*  InputSameDT=on  SaturateOnIntegerOverflow=on  OutDataTypeStr=Inherit: Same as first input
  Product5 : Product  Inputs=/*  InputSameDT=on  SaturateOnIntegerOverflow=on  OutDataTypeStr=Inherit: Same as first input
  Real-Imag to Complex1 : RealImagToComplex
  Real-Imag to Complex2 : RealImagToComplex
  Real-Imag to Complex5 : RealImagToComplex
  Selector1 : Selector  InputPortWidth=3  IndexOptions=Index vector (dialog)  Indices=1  OutputSizes=1
  Selector2 : Selector  InputPortWidth=3  IndexOptions=Index vector (dialog)  Indices=1  OutputSizes=1
  Selector6 : Selector  InputPortWidth=3  IndexOptions=Index vector (dialog)  Indices=1  OutputSizes=1
  Series RLC Branch10 : spsSeriesRLCBranchLib/Series RLC Branch  LConnTagsString=__new0  RConnTagsString=__new0  BranchType=R  Resistance=1e12  Inductance=1e-3  SetiL0=off  InitialCurrent=0  Capacitance=1e-6  Setx0=off  InitialVoltage=0  Measurements=None
  Series RLC Branch11 : spsSeriesRLCBranchLib/Series RLC Branch  LConnTagsString=__new0  RConnTagsString=__new0  BranchType=R  Resistance=1e12  Inductance=1e-3  SetiL0=off  InitialCurrent=0  Capacitance=1e-6  Setx0=off  InitialVoltage=0  Measurements=None
  Series RLC Branch9 : spsSeriesRLCBranchLib/Series RLC Branch  LConnTagsString=__new0  RConnTagsString=__new0  BranchType=R  Resistance=1e12  Inductance=1e-3  SetiL0=off  InitialCurrent=0  Capacitance=1e-6  Setx0=off  InitialVoltage=0  Measurements=None
  Three-Phase Sine Generator : spsThreePhaseSineGeneratorLib/Three-Phase Sine Generator  Ts=0
      settings: LibrarySourceBlock=|
      | sps_lib/Sources/Signal Generator Sources/Three-Phase
      | Sine Generator
  Three-Phase Sine Generator1 : spsThreePhaseSineGeneratorLib/Three-Phase Sine Generator  Ts=0
      settings: LibrarySourceBlock=|
      | sps_lib/Sources/Signal Generator Sources/Three-Phase
      | Sine Generator
  Three-Phase Sine Generator2 : spsThreePhaseSineGeneratorLib/Three-Phase Sine Generator  Ts=0
      settings: LibrarySourceBlock=|
      | sps_lib/Sources/Signal Generator Sources/Three-Phase
      | Sine Generator
  Three-Phase V-I Measurement1 : spsThreePhaseVIMeasurementLib/Three-Phase V-I Measurement  VoltageMeasurement=phase-to-phase  SetLabelV=off  LabelV=Vabc  Vpu=off  VpuLL=off  CurrentMeasurement=yes  SetLabelI=off  LabelI=Iabc  Ipu=off  Pbase=100e6  Vbase=Vnom*sqrt(3)  OutputType=Complex  PhasorSimulation=off  PSBequivalent=0
  To Workspace2 : ToWorkspace  Commented=on  VariableName=I_RMS_3ph_nsec  SampleTime=timestep_meas_data * t_factor
  To Workspace4 : ToWorkspace  Commented=on  VariableName=I_RMS_3ph_0_1sec  SampleTime=0.1 * t_factor
  To Workspace5 : ToWorkspace  Commented=on  VariableName=I_RMS_3ph_1sec  SampleTime=1 * t_factor
  "TrueRMS " : Subsystem  AncestorBlock=powerlib_meascontrol/Measurements/RMS/TrueRMS
  TrueRMS 1 : Subsystem  Commented=on  AncestorBlock=powerlib_meascontrol/Measurements/RMS/TrueRMS
  Unit Delay4 : UnitDelay  InitialCondition=0*exp(-j*0*pi/180)  SampleTime=Ts  HasFrameUpgradeWarning=on
  L1 : PMIOPort  Side=Right
  L2 : PMIOPort  Port=2  Side=Right
  L3 : PMIOPort  Port=3  Side=Right
  wires:
  1-D AP_L1/1 -> Mux1/1
  Product5/1 -> Conj4/1
  Three-Phase V-I Measurement1/2 -> Goto/1, TrueRMS 1/1(In)
  Mux1/1 -> Demux1/1
  Real-Imag to Complex5/1 -> Product5/2
  Clock7/1 -> 1-D RP_L1/1, 1-D RP_L2/1, 1-D AP_L3/1, 1-D RP_L3/1, 1-D AP_L2/1, 1-D AP_L1/1
  TrueRMS 1/1(RMS) -> To Workspace2/1, To Workspace5/1, To Workspace4/1
  Constant/1 -> Magnitude-Angle to Complex/2
  Demux/1 -> Product5/1
  Demux/2 -> Product2/1
  Demux/3 -> Product4/1
  Magnitude-Angle to Complex/1 -> Demux/1
  Gain/1 -> Magnitude-Angle to Complex/1
  Mux/1 -> Unit Delay4/1
  Complex to Magnitude-Angle/1 -> Gain1/1
  Three-Phase Sine Generator/1 -> Selector1/1
  Three-Phase Sine Generator1/1 -> Selector2/1
  Three-Phase Sine Generator2/1 -> Selector6/1
  Selector2/1 -> Controlled Current Source4/1
  Selector6/1 -> Controlled Current Source5/1
  Demux2/1 -> Three-Phase Sine Generator/1
  Demux2/2 -> Three-Phase Sine Generator1/1
  Demux2/3 -> Three-Phase Sine Generator2/1
  Conj4/1 -> Mux/1
  Conj1/1 -> Mux/2
  Conj2/1 -> Mux/3
  Constant1/1 -> Three-Phase Sine Generator/3, Three-Phase Sine Generator2/3, Three-Phase Sine Generator1/3
  Complex to Magnitude-Angle/2 -> Gain3/1
  Gain3/1 -> Demux4/1
  Selector1/1 -> Controlled Current Source3/1
  Demux4/1 -> Three-Phase Sine Generator/2
  Demux4/2 -> Three-Phase Sine Generator1/2
  Demux4/3 -> Three-Phase Sine Generator2/2
  Gain1/1 -> Demux2/1
  Demux1/1 -> Real-Imag to Complex5/1
  Demux1/2 -> Real-Imag to Complex5/2
  "TrueRMS "/1(RMS) -> Gain/1
  Three-Phase V-I Measurement1/1 -> "TrueRMS "/1(In)
  Unit Delay4/1 -> Complex to Magnitude-Angle/1
  Mux2/1 -> Demux3/1
  Demux3/2 -> Real-Imag to Complex1/2
  Real-Imag to Complex1/1 -> Product2/2
  Demux3/1 -> Real-Imag to Complex1/1
  1-D AP_L2/1 -> Mux2/1
  Product2/1 -> Conj1/1
  Mux4/1 -> Demux5/1
  Demux5/2 -> Real-Imag to Complex2/2
  Real-Imag to Complex2/1 -> Product4/2
  Demux5/1 -> Real-Imag to Complex2/1
  1-D AP_L3/1 -> Mux4/1
  Product4/1 -> Conj2/1
  1-D RP_L1/1 -> Mux1/2
  1-D RP_L2/1 -> Mux2/2
  1-D RP_L3/1 -> Mux4/2
  connections:
  Three-Phase V-I Measurement1/RConn2 -- Controlled Current Source4/LConn1
  Three-Phase V-I Measurement1/RConn1 -- Controlled Current Source3/LConn1
  Three-Phase V-I Measurement1/RConn3 -- Controlled Current Source5/LConn1
  Controlled Current Source3/RConn1 -- Controlled Current Source4/RConn1 -- Ground8/LConn1 -- Controlled Current Source5/RConn1
  L1/RConn1 -- Three-Phase V-I Measurement1/LConn1 -- Series RLC Branch9/LConn1
  Series RLC Branch10/LConn1 -- Three-Phase V-I Measurement1/LConn2 -- L2/RConn1
  Series RLC Branch11/LConn1 -- Three-Phase V-I Measurement1/LConn3 -- L3/RConn1
  Series RLC Branch9/RConn1 -- Series RLC Branch10/RConn1 -- Ground3/LConn1 -- Series RLC Branch11/RConn1

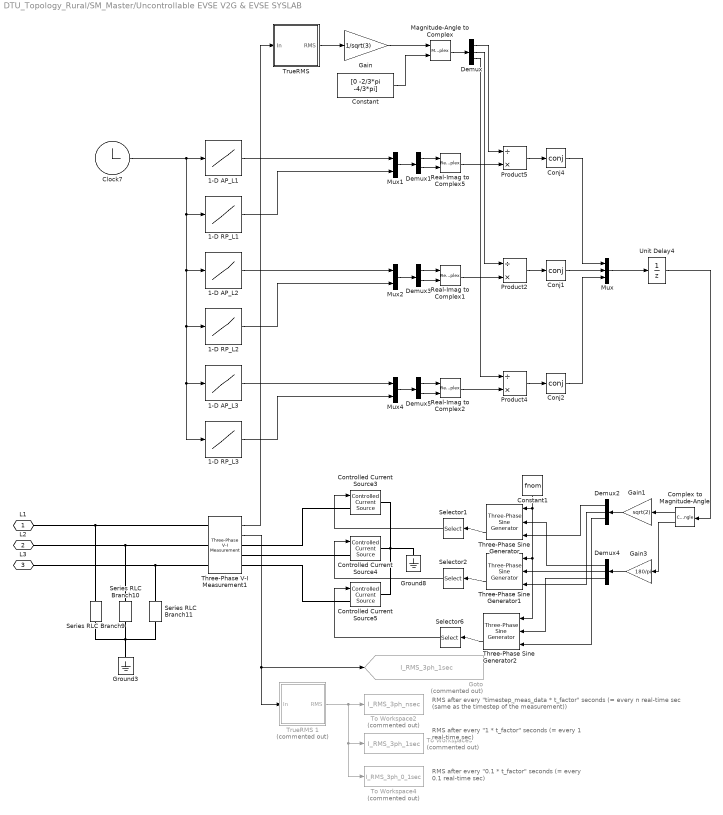
== system DTU_Topology_Rural/SM_Master/Uncontrollable EVSE V2G & EVSE SYSLAB ==
  note: RMS after every "1 * t_factor" seconds
      | (= every 1 real-time sec)
  note: RMS after every "0.1 * t_factor" seconds
      | (= every 0.1 real-time sec)
  note: RMS after every "timestep_meas_data * t_factor" seconds
      | (= every n real-time sec (same as the timestep of the measurement))
  1-D AP_L1 : Lookup_n-D  NumberOfTableDimensions=1  BreakpointsForDimension1=Time  Table="data.(\"319-3_B2 to 715-2_phaseA_ActivePower\")(datastart:datastop) * DTUsignconv"  InterpMethod=Flat  InternalRulePriority=Speed  RndMeth=Simplest
  1-D AP_L2 : Lookup_n-D  NumberOfTableDimensions=1  BreakpointsForDimension1=Time  Table="data.(\"319-3_B2 to 715-2_phaseB_ActivePower\")(datastart:datastop) * DTUsignconv"  InterpMethod=Flat  InternalRulePriority=Speed  RndMeth=Simplest
  1-D AP_L3 : Lookup_n-D  NumberOfTableDimensions=1  BreakpointsForDimension1=Time  Table="data.(\"319-3_B2 to 715-2_phaseC_ActivePower\")(datastart:datastop) * DTUsignconv"  InterpMethod=Flat  InternalRulePriority=Speed  RndMeth=Simplest
  1-D RP_L1 : Lookup_n-D  NumberOfTableDimensions=1  BreakpointsForDimension1=Time  Table="data.(\"319-3_B2 to 715-2_phaseA_ReactivePower\")(datastart:datastop) * DTUsignconv"  InterpMethod=Flat  InternalRulePriority=Speed  RndMeth=Simplest
  1-D RP_L2 : Lookup_n-D  NumberOfTableDimensions=1  BreakpointsForDimension1=Time  Table="data.(\"319-3_B2 to 715-2_phaseB_ReactivePower\")(datastart:datastop) * DTUsignconv"  InterpMethod=Flat  InternalRulePriority=Speed  RndMeth=Simplest
  1-D RP_L3 : Lookup_n-D  NumberOfTableDimensions=1  BreakpointsForDimension1=Time  Table="data.(\"319-3_B2 to 715-2_phaseC_ReactivePower\")(datastart:datastop) * DTUsignconv"  InterpMethod=Flat  InternalRulePriority=Speed  RndMeth=Simplest
  Clock7 : Clock
  Complex to Magnitude-Angle : ComplexToMagnitudeAngle
  Conj1 : Math  Operator=conj  SignedPower=on
  Conj2 : Math  Operator=conj  SignedPower=on
  Conj4 : Math  Operator=conj  SignedPower=on
  Constant : Constant  Value=[0 -2/3*pi -4/3*pi]
  Constant1 : Constant  Value=fnom
  Controlled Current Source3 : spsControlledCurrentSourceLib/Controlled Current Source  Initialize=on  Source_Type=AC  Amplitude=0  Phase=0  Frequency=50  Measurements=Current
  Controlled Current Source4 : spsControlledCurrentSourceLib/Controlled Current Source  Initialize=on  Source_Type=AC  Amplitude=0  Phase=0  Frequency=50  Measurements=Current
  Controlled Current Source5 : spsControlledCurrentSourceLib/Controlled Current Source  Initialize=on  Source_Type=AC  Amplitude=0  Phase=0  Frequency=50  Measurements=Current
  Demux : Demux  Outputs=3
  Demux1 : Demux  Outputs=2
      settings: DisplayOption=none
  Demux2 : Demux  Outputs=3
  Demux3 : Demux  Outputs=2
      settings: DisplayOption=none
  Demux4 : Demux  Outputs=3
  Demux5 : Demux  Outputs=2
      settings: DisplayOption=none
  Gain : Gain  Gain=1/sqrt(3)
  Gain1 : Gain  Gain=sqrt(2)
  Gain3 : Gain  Gain=180/pi
  Goto : Goto  Commented=on  GotoTag=I_RMS_3ph_1sec  TagVisibility=global
  Ground3 : spsGroundLib/Ground  LConnTagsString=a
  Ground8 : spsGroundLib/Ground  LConnTagsString=a
  Magnitude-Angle to Complex : MagnitudeAngleToComplex
  Mux : Mux  Inputs=3
  Mux1 : Mux  Inputs=2
  Mux2 : Mux  Inputs=2
  Mux4 : Mux  Inputs=2
  Product2 : Product  Inputs=/*  InputSameDT=on  SaturateOnIntegerOverflow=on  OutDataTypeStr=Inherit: Same as first input
  Product4 : Product  Inputs=/*  InputSameDT=on  SaturateOnIntegerOverflow=on  OutDataTypeStr=Inherit: Same as first input
  Product5 : Product  Inputs=/*  InputSameDT=on  SaturateOnIntegerOverflow=on  OutDataTypeStr=Inherit: Same as first input
  Real-Imag to Complex1 : RealImagToComplex
  Real-Imag to Complex2 : RealImagToComplex
  Real-Imag to Complex5 : RealImagToComplex
  Selector1 : Selector  InputPortWidth=3  IndexOptions=Index vector (dialog)  Indices=1  OutputSizes=1
  Selector2 : Selector  InputPortWidth=3  IndexOptions=Index vector (dialog)  Indices=1  OutputSizes=1
  Selector6 : Selector  InputPortWidth=3  IndexOptions=Index vector (dialog)  Indices=1  OutputSizes=1
  Series RLC Branch10 : spsSeriesRLCBranchLib/Series RLC Branch  LConnTagsString=__new0  RConnTagsString=__new0  BranchType=R  Resistance=1e12  Inductance=1e-3  SetiL0=off  InitialCurrent=0  Capacitance=1e-6  Setx0=off  InitialVoltage=0  Measurements=None
  Series RLC Branch11 : spsSeriesRLCBranchLib/Series RLC Branch  LConnTagsString=__new0  RConnTagsString=__new0  BranchType=R  Resistance=1e12  Inductance=1e-3  SetiL0=off  InitialCurrent=0  Capacitance=1e-6  Setx0=off  InitialVoltage=0  Measurements=None
  Series RLC Branch9 : spsSeriesRLCBranchLib/Series RLC Branch  LConnTagsString=__new0  RConnTagsString=__new0  BranchType=R  Resistance=1e12  Inductance=1e-3  SetiL0=off  InitialCurrent=0  Capacitance=1e-6  Setx0=off  InitialVoltage=0  Measurements=None
  Three-Phase Sine Generator : spsThreePhaseSineGeneratorLib/Three-Phase Sine Generator  Ts=0
      settings: LibrarySourceBlock=|
      | sps_lib/Sources/Signal Generator Sources/Three-Phase
      | Sine Generator
  Three-Phase Sine Generator1 : spsThreePhaseSineGeneratorLib/Three-Phase Sine Generator  Ts=0
      settings: LibrarySourceBlock=|
      | sps_lib/Sources/Signal Generator Sources/Three-Phase
      | Sine Generator
  Three-Phase Sine Generator2 : spsThreePhaseSineGeneratorLib/Three-Phase Sine Generator  Ts=0
      settings: LibrarySourceBlock=|
      | sps_lib/Sources/Signal Generator Sources/Three-Phase
      | Sine Generator
  Three-Phase V-I Measurement1 : spsThreePhaseVIMeasurementLib/Three-Phase V-I Measurement  VoltageMeasurement=phase-to-phase  SetLabelV=off  LabelV=Vabc  Vpu=off  VpuLL=off  CurrentMeasurement=yes  SetLabelI=off  LabelI=Iabc  Ipu=off  Pbase=100e6  Vbase=Vnom*sqrt(3)  OutputType=Complex  PhasorSimulation=off  PSBequivalent=0
  To Workspace2 : ToWorkspace  Commented=on  VariableName=I_RMS_3ph_nsec  SampleTime=timestep_meas_data * t_factor
  To Workspace4 : ToWorkspace  Commented=on  VariableName=I_RMS_3ph_0_1sec  SampleTime=0.1 * t_factor
  To Workspace5 : ToWorkspace  Commented=on  VariableName=I_RMS_3ph_1sec  SampleTime=1 * t_factor
  "TrueRMS " : Subsystem  AncestorBlock=powerlib_meascontrol/Measurements/RMS/TrueRMS
  TrueRMS 1 : Subsystem  Commented=on  AncestorBlock=powerlib_meascontrol/Measurements/RMS/TrueRMS
  Unit Delay4 : UnitDelay  InitialCondition=0*exp(-j*0*pi/180)  SampleTime=Ts  HasFrameUpgradeWarning=on
  L1 : PMIOPort  Side=Right
  L2 : PMIOPort  Port=2  Side=Right
  L3 : PMIOPort  Port=3  Side=Right
  wires:
  1-D AP_L1/1 -> Mux1/1
  Product5/1 -> Conj4/1
  Three-Phase V-I Measurement1/2 -> Goto/1, TrueRMS 1/1(In)
  Mux1/1 -> Demux1/1
  Real-Imag to Complex5/1 -> Product5/2
  Clock7/1 -> 1-D RP_L1/1, 1-D RP_L2/1, 1-D AP_L3/1, 1-D RP_L3/1, 1-D AP_L2/1, 1-D AP_L1/1
  TrueRMS 1/1(RMS) -> To Workspace2/1, To Workspace5/1, To Workspace4/1
  Constant/1 -> Magnitude-Angle to Complex/2
  Demux/1 -> Product5/1
  Demux/2 -> Product2/1
  Demux/3 -> Product4/1
  Magnitude-Angle to Complex/1 -> Demux/1
  Gain/1 -> Magnitude-Angle to Complex/1
  Mux/1 -> Unit Delay4/1
  Complex to Magnitude-Angle/1 -> Gain1/1
  Three-Phase Sine Generator/1 -> Selector1/1
  Three-Phase Sine Generator1/1 -> Selector2/1
  Three-Phase Sine Generator2/1 -> Selector6/1
  Selector2/1 -> Controlled Current Source4/1
  Selector6/1 -> Controlled Current Source5/1
  Demux2/1 -> Three-Phase Sine Generator/1
  Demux2/2 -> Three-Phase Sine Generator1/1
  Demux2/3 -> Three-Phase Sine Generator2/1
  Conj4/1 -> Mux/1
  Conj1/1 -> Mux/2
  Conj2/1 -> Mux/3
  Constant1/1 -> Three-Phase Sine Generator/3, Three-Phase Sine Generator2/3, Three-Phase Sine Generator1/3
  Complex to Magnitude-Angle/2 -> Gain3/1
  Gain3/1 -> Demux4/1
  Selector1/1 -> Controlled Current Source3/1
  Demux4/1 -> Three-Phase Sine Generator/2
  Demux4/2 -> Three-Phase Sine Generator1/2
  Demux4/3 -> Three-Phase Sine Generator2/2
  Gain1/1 -> Demux2/1
  Demux1/1 -> Real-Imag to Complex5/1
  Demux1/2 -> Real-Imag to Complex5/2
  "TrueRMS "/1(RMS) -> Gain/1
  Three-Phase V-I Measurement1/1 -> "TrueRMS "/1(In)
  Unit Delay4/1 -> Complex to Magnitude-Angle/1
  Mux2/1 -> Demux3/1
  Demux3/2 -> Real-Imag to Complex1/2
  Real-Imag to Complex1/1 -> Product2/2
  Demux3/1 -> Real-Imag to Complex1/1
  1-D AP_L2/1 -> Mux2/1
  Product2/1 -> Conj1/1
  Mux4/1 -> Demux5/1
  Demux5/2 -> Real-Imag to Complex2/2
  Real-Imag to Complex2/1 -> Product4/2
  Demux5/1 -> Real-Imag to Complex2/1
  1-D AP_L3/1 -> Mux4/1
  Product4/1 -> Conj2/1
  1-D RP_L1/1 -> Mux1/2
  1-D RP_L2/1 -> Mux2/2
  1-D RP_L3/1 -> Mux4/2
  connections:
  Three-Phase V-I Measurement1/RConn2 -- Controlled Current Source4/LConn1
  Three-Phase V-I Measurement1/RConn1 -- Controlled Current Source3/LConn1
  Three-Phase V-I Measurement1/RConn3 -- Controlled Current Source5/LConn1
  Controlled Current Source3/RConn1 -- Controlled Current Source4/RConn1 -- Ground8/LConn1 -- Controlled Current Source5/RConn1
  L1/RConn1 -- Three-Phase V-I Measurement1/LConn1 -- Series RLC Branch9/LConn1
  Series RLC Branch10/LConn1 -- Three-Phase V-I Measurement1/LConn2 -- L2/RConn1
  Series RLC Branch11/LConn1 -- Three-Phase V-I Measurement1/LConn3 -- L3/RConn1
  Series RLC Branch9/RConn1 -- Series RLC Branch10/RConn1 -- Ground3/LConn1 -- Series RLC Branch11/RConn1
